simulink model "MPC_traj"  (R2015a)
settings: Solver=ode4  StartTime=0.0  StopTime=10  FixedStep=0.01  RelTol=1e-3
settings Model: Creator=LAB425  LastModifiedBy=LAB425

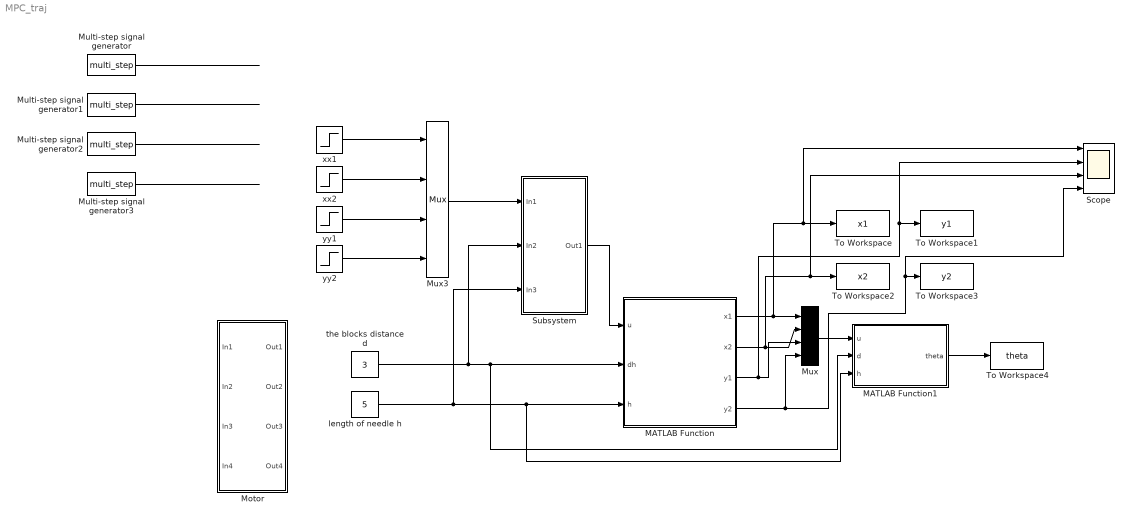
== system MPC_traj ==
  MATLAB Function : MATLAB Function  TreatAsAtomicUnit=on
  MATLAB Function1 : MATLAB Function  TreatAsAtomicUnit=on
  "Motor " : Subsystem
  Multi-step signal generator : S-Function  FunctionName=multi_step  Parameters=tTime,yStep  mask{tTime=[0,5], yStep=[-2,-1]}
      mask prompts: tTime "Time instances"; yStep "Step Values"
      mask init:
      | xx=repmat(tTime,2,1); yy=repmat(yStep,2,1);
      | xx=[xx(:)' 2*tTime(end)-tTime(end-1)];
      | yy=[0, yy(:)'];
      mask Display: plot(xx,yy)
  Multi-step signal generator1 : S-Function  FunctionName=multi_step  Parameters=tTime,yStep  mask{tTime=[0,5], yStep=[0.5,0]}
      mask prompts: tTime "Time instances"; yStep "Step Values"
      mask init:
      | xx=repmat(tTime,2,1); yy=repmat(yStep,2,1);
      | xx=[xx(:)' 2*tTime(end)-tTime(end-1)];
      | yy=[0, yy(:)'];
      mask Display: plot(xx,yy)
  Multi-step signal generator2 : S-Function  FunctionName=multi_step  Parameters=tTime,yStep  mask{tTime=[0,5], yStep=[-2,0]}
      mask prompts: tTime "Time instances"; yStep "Step Values"
      mask init:
      | xx=repmat(tTime,2,1); yy=repmat(yStep,2,1);
      | xx=[xx(:)' 2*tTime(end)-tTime(end-1)];
      | yy=[0, yy(:)'];
      mask Display: plot(xx,yy)
  Multi-step signal generator3 : S-Function  FunctionName=multi_step  Parameters=tTime,yStep  mask{tTime=[0,5], yStep=[1,0]}
      mask prompts: tTime "Time instances"; yStep "Step Values"
      mask init:
      | xx=repmat(tTime,2,1); yy=repmat(yStep,2,1);
      | xx=[xx(:)' 2*tTime(end)-tTime(end-1)];
      | yy=[0, yy(:)'];
      mask Display: plot(xx,yy)
  Mux : Mux
  Mux3 : Mux
  Scope : Scope  NumInputPorts=4
      settings: TimeRange=10  YMin=-5~-5~-5~-5  YMax=5~5~5~5
  Subsystem : Subsystem
  To Workspace : ToWorkspace  VariableName=x1  SaveFormat=Timeseries  SampleTime=-1
  To Workspace1 : ToWorkspace  VariableName=y1  SaveFormat=Timeseries  SampleTime=-1
  To Workspace2 : ToWorkspace  VariableName=x2  SaveFormat=Timeseries  SampleTime=-1
  To Workspace3 : ToWorkspace  VariableName=y2  SaveFormat=Timeseries  SampleTime=-1
  To Workspace4 : ToWorkspace  VariableName=theta  SaveFormat=Timeseries  SampleTime=-1
  length of needle h : Constant  Value=5
  the blocks distance d : Constant  Value=3
  xx1 : Step  Time=0  Before=-2  After=-2
  xx2 : Step  Time=0  Before=0.5  After=0.5
  yy1 : Step  Time=0  Before=-2  After=-2
  yy2 : Step  Time=5  Before=1
  wires:
  the blocks distance d/1 -> MATLAB Function1/2(d), MATLAB Function/2(dh), Subsystem/2(In2)
  length of needle h/1 -> Subsystem/3(In3), MATLAB Function1/3(h), MATLAB Function/3(h)
  Subsystem/1(Out1) -> MATLAB Function/1(u)
  MATLAB Function/2(x2) -> Scope/3, To Workspace2/1, Mux/2
  Mux/1 -> MATLAB Function1/1(u)
  MATLAB Function1/1(theta) -> To Workspace4/1
  MATLAB Function/1(x1) -> Scope/1, To Workspace/1, Mux/1
  MATLAB Function/3(y1) -> To Workspace1/1, Scope/2, Mux/3
  MATLAB Function/4(y2) -> Mux/4, To Workspace3/1, Scope/4
  Mux3/1 -> Subsystem/1(In1)
  Multi-step signal generator/1 -> ?
  Multi-step signal generator1/1 -> ?
  Multi-step signal generator2/1 -> ?
  Multi-step signal generator3/1 -> ?
  xx1/1 -> Mux3/1
  xx2/1 -> Mux3/2
  yy1/1 -> Mux3/3
  yy2/1 -> Mux3/4

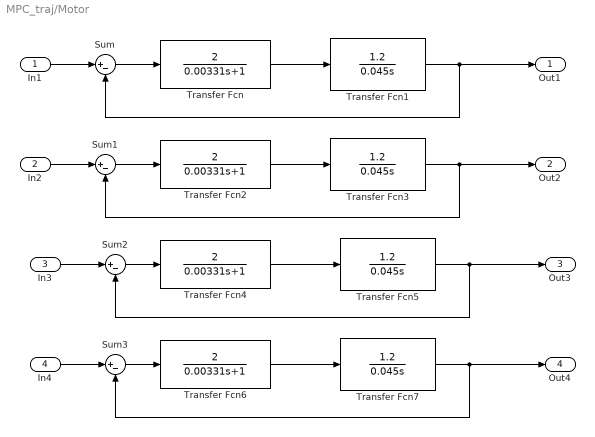
== system MPC_traj/Motor  ==
  In1 : Inport
  In2 : Inport  Port=2
  In3 : Inport  Port=3
  In4 : Inport  Port=4
  Sum{,1..3} (4 alike) : Sum  Inputs=|+-
  Transfer Fcn{,2,4,6} (4 alike) : TransferFcn  Numerator=[2]  Denominator=[0.00331 1]
  Transfer Fcn{1,3,5,7} (4 alike) : TransferFcn  Numerator=[1.2]  Denominator=[0.045 0]
  Out1 : Outport
  Out2 : Outport  Port=2
  Out3 : Outport  Port=3
  Out4 : Outport  Port=4
  wires:
  Transfer Fcn1/1 -> Out1/1, Sum/2
  In1/1 -> Sum/1
  Transfer Fcn/1 -> Transfer Fcn1/1
  Sum/1 -> Transfer Fcn/1
  Transfer Fcn3/1 -> Out2/1, Sum1/2
  In2/1 -> Sum1/1
  Transfer Fcn2/1 -> Transfer Fcn3/1
  Sum1/1 -> Transfer Fcn2/1
  Transfer Fcn5/1 -> Out3/1, Sum2/2
  In3/1 -> Sum2/1
  Transfer Fcn4/1 -> Transfer Fcn5/1
  Sum2/1 -> Transfer Fcn4/1
  Transfer Fcn7/1 -> Out4/1, Sum3/2
  In4/1 -> Sum3/1
  Transfer Fcn6/1 -> Transfer Fcn7/1
  Sum3/1 -> Transfer Fcn6/1

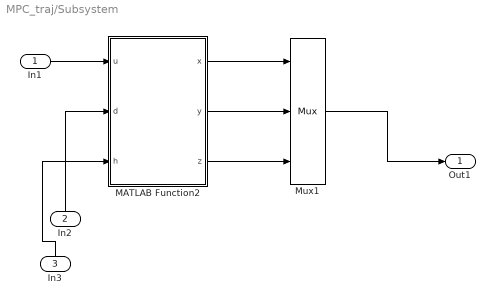
== system MPC_traj/Subsystem ==
  In1 : Inport
  In2 : Inport  Port=2
  In3 : Inport  Port=3
  MATLAB Function2 : MATLAB Function  TreatAsAtomicUnit=on
  Mux1 : Mux  Inputs=3
  Out1 : Outport
  wires:
  MATLAB Function2/1(x) -> Mux1/1
  MATLAB Function2/2(y) -> Mux1/2
  Mux1/1 -> Out1/1
  MATLAB Function2/3(z) -> Mux1/3
  In1/1 -> MATLAB Function2/1(u)
  In2/1 -> MATLAB Function2/2(d)
  In3/1 -> MATLAB Function2/3(h)

== matlab function MPC_traj/MATLAB Function1 ==
  data: u input; d input; h input; theta output
function theta  = get_theta(u,d,h)
%#codegen

% y = u;
% mid = asin(u/5);
% 
% mid2 = 3 * tan(mid);
% 
% ymid = mid2 / 0.2;
% 
% y = pi * ymid;

x1 = u(1);x2 = u(2);y1 = u(3); y2 = u(4);

% T01=[1,0,0,0;0,cos(atan2((x1+x2),d)),-sin(atan2((x1+x2),d)),0;0,sin(atan2((x1+x2),d)),cos(atan2((x1+x2),d)),x1;0,0,0,1];
% T1m=[0,0,1,0;1,0,0,0,;0,1,0,0;0,0,0,1];
% Tmm1=[0,1,0,0;-1,0,0,0;0,0,1,0;0,0,0,1];
% Tm12=[1,0,0,0;0,cos(atan2((y1+y2),d))];
forwardx = sign(x1);forwardy = sign(y1);

X = abs(x1) + abs(x2);
Y = abs(y1) + abs(y2);
L = sqrt(X^2+Y^2);
theta = atan2(L,d);
H = h * sin(theta);
z = -h * cos(theta);
beta = atan2(Y,X);
y = -forwardy * (H * sin(beta) + abs(y2));
x = -forwardx * (H * cos(beta) + abs(x2));

== matlab function MPC_traj/MATLAB Function ==
  data: u input; x1 output; dh input; h input; x2 output; y1 output; y2 output
function [x1,x2,y1,y2] = inv(u,dh,h)
%#codegen
% u = 2.5
% y = u;
limit = 2.774;
X=u(1);Y=u(2);Z=u(3);
forwardx = sign(X);forwardy=sign(Y);

if (-limit<= X && X <= limit) && (-limit<= Y && Y <= limit)
    X=abs(X);Y=abs(Y);
    beta = atan2(Y,X);
    H=sqrt(X^2+Y^2);
    theta=asin(H/h);
    D=dh*tan(theta);
    y1 = -forwardy * D * sin(beta);
    x1 = -forwardx * D * cos(beta);
    x2 = 0;
    y2 = 0;
else
    y1 = -forwardy * 2;x1 = -forwardx * 2;
    a = x1; 
    b = y1;
    d = Y; 
    c = X;
    B = h^2 - Z^2;
    D = real((dh * tan(acos(complex(abs(Z)/h)))))^2;
    E = (B - D - c^2 + a^2 - d^2 + b^2) / 2 ;
    F = a - c;
    G = b - d;
   
    EA = (F^2 + G^2)/G^2;
    EB = (2*G*d*F - 2*G^2*c - 2*E*F)/G^2;
    EC = (G^2*c^2 + G^2*d^2 - 2*G*d*E + E^2 - B*G^2)/G^2;
%     if (EB^2 - 4*EA*EC) < 0
%          y1 = -forwardy * 2;x1 = -forwardx * 2;
%          y2 = forwardy * 2;x2 = forwardx * 2;
    if sign((-EB + real(sqrt(complex(EB^2 - 4*EA*EC)))) / (2*EA)) == sign(forwardx)
        x2 = (-EB + real(sqrt(complex(EB^2 - 4*EA*EC)))) / (2*EA);
        y2 = (E - F*x2) / G;
    else
        x2 = (-EB - real(sqrt(complex(EB^2 - 4*EA*EC)))) / (2*EA);
        y2 = (E - F*x2) / G;
    end
end
%     X = abs(x1) + abs(x2);
%     Y = abs(y1) + abs(y2);
%     L = sqrt(X^2+Y^2);
%     theta = atan2(L,d);
%     H = h * sin(theta);
%     z = -h * cos(theta);
%     beta = atan2(Y,X);
%     y = -forwardy * (H * sin(beta) + abs(y2));
%     x = -forwardx * (H * cos(beta) + abs(x2));



% %     E = B - D - x^2 + x1^2 - y^2 + y1^2;
% %     F = 2*y1 + 2*y;
% %     G = 2*x1 + 2*x;
% %     A = F^2 + G^2;
% %     BB = 2*F*y1*G - 2*F^2*x1 - 2*E*G;
% %     C = F^2*x1^2 + F*y1^2 - 2*F*y1*E + E^2 - D*F^2;
% %     if (BB^2 - 4*A*C) < 0
% %         y1 = -forwardy * 2;x1 = -forwardx * 2;
% %         y2 = forwardy * 2;x2 = forwardx * 2;
% %     elseif (sign((-BB-sqrt(BB^2-4*A*C))/2*A) == sign(forwardx)) && ((-BB-sqrt(BB^2-4*A*C))/2*A <= 2) && ((-B-sqrt(B^2-4*A*C))/2*A >= -2)
% %         y1 = -forwardy * 2;x1 = -forwardx * 2;
% %         x2 = (-BB-sqrt(BB^2-4*A*C))/2*A;
% %         y2 = (E - G*x2)/F;
% %     else
% %         y1 = -forwardy * 2;x1 = -forwardx * 2;
% %         x2 = (-BB+sqrt(BB^2-4*A*C))/2*A;
% %         y2 = (E - G*x2)/F;
% %     end
%     A = (D-B+d^2+c^2-a^2-b^2)/2;
%     AA=(b-c)^2+(d-a)^2;
%     BB=2*A*(b-c)-2*b*(d-a)^2-2*a*(A+(b-c))*(d-a);
%     CC=A^2-(D-a^2-b^2)*(d-a)^2
% %     if (B^2 - 4*A*C) < 0
% %         y1 = -forwardy * 2;x1 = -forwardx * 2;
% %         y2 = forwardy * 2;x2 = forwardx * 2;
% %     elseif (sign((-B-sqrt(B^2-4*A*C))/2*A) == sign(forwardx)) && ((-B-sqrt(B^2-4*A*C))/2*A <= 2) && ((-B-sqrt(B^2-4*A*C))/2*A >= -2)
% %         y1 = -forwardy * 2;x1 = -forwardx * 2;
% %         x2 = (-B-sqrt(B^2-4*A*C))/2*A;
% %         y2 = 0;
% %     else
% %         y1 = -forwardy * 2;x1 = -forwardx * 2;
% %         x2 = (-B+sqrt(B^2-4*A*C))/2*A;
% %         y2 = 0;
% %     end
%      y1 = -forwardy * 2;x1 = -forwardx * 2;
%      x2 = (-BB + sqrt(BB^2 - 4 * AA * CC)) / 2 * AA;
%      y2=0;
end

== matlab function MPC_traj/Subsystem/MATLAB Function2 ==
  data: x output; u input; y output; z output; d input; h input
function [x,y,z] = forward(u,d,h)
%#codegen

% y = u;
% mid = asin(u/5);
% 
% mid2 = 3 * tan(mid);
% 
% ymid = mid2 / 0.2;
% 
% y = pi * ymid;

x1 = u(1);x2 = u(2);y1 = u(3); y2 = u(4);

% T01=[1,0,0,0;0,cos(atan2((x1+x2),d)),-sin(atan2((x1+x2),d)),0;0,sin(atan2((x1+x2),d)),cos(atan2((x1+x2),d)),x1;0,0,0,1];
% T1m=[0,0,1,0;1,0,0,0,;0,1,0,0;0,0,0,1];
% Tmm1=[0,1,0,0;-1,0,0,0;0,0,1,0;0,0,0,1];
% Tm12=[1,0,0,0;0,cos(atan2((y1+y2),d))];
forwardx = sign(x1);forwardy = sign(y1);

X = abs(x1) + abs(x2);
Y = abs(y1) + abs(y2);
L = sqrt(X^2+Y^2);
theta = atan2(L,d);
H = h * sin(theta);
z = -h * cos(theta);
beta = atan2(Y,X);
y = -forwardy * (H * sin(beta) + abs(y2));
x = -forwardx * (H * cos(beta) + abs(x2));
